simulink model "zaw_int"  (R2013a)
settings: Solver=ode3  StartTime=0.0  StopTime=10.0  FixedStep=0.005  RelTol=1e-3
values from neighbouring files (symbols this model uses):
  c1 = 100    [matlab.mat]    (also in matlab1.mat; matlab3.mat; matlab4.mat)
  c2 = 2000    [matlab.mat]    (also in matlab1.mat; matlab3.mat; matlab4.mat)
  k1 = 370000    [matlab.mat]    (also in matlab1.mat; matlab3.mat; matlab4.mat)
  k2 = 35000    [matlab.mat]    (also in matlab1.mat; matlab3.mat; matlab4.mat = 15000)
  m1 = 90    [matlab.mat]    (also in matlab1.mat; matlab3.mat; matlab4.mat)
  m2 = 600    [matlab.mat]    (also in matlab1.mat; matlab3.mat; matlab4.mat)
  T1 = 0.88    [matlab3.mat]    (also in matlab4.mat)
settings Model: Creator=adasdeb  LastModifiedBy=adasdeb

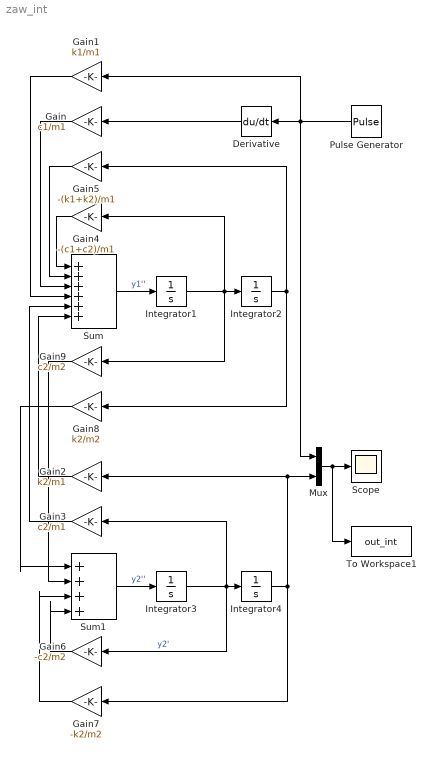
== system zaw_int ==
  Derivative : Derivative
  Gain : Gain  Gain=c1/m1
  Gain1 : Gain  Gain=k1/m1
  Gain2 : Gain  Gain=k2/m1
  Gain3 : Gain  Gain=c2/m1
  Gain4 : Gain  Gain=-(c1+c2)/m1
  Gain5 : Gain  Gain=-(k1+k2)/m1
  Gain6 : Gain  Gain=-c2/m2
  Gain7 : Gain  Gain=-k2/m2
  Gain8 : Gain  Gain=k2/m2
  Gain9 : Gain  Gain=c2/m2
  Integrator{1..4} (4 alike) : Integrator
  Mux : Mux  Inputs=2
  Pulse Generator : DiscretePulseGenerator  PulseType=Time based  Period=T1  PulseWidth=50
  Scope : Scope
      settings: YMin=-2  YMax=2
  Sum : Sum  Inputs=|++++++|
  Sum1 : Sum  Inputs=|++++|
  To Workspace1 : ToWorkspace  VariableName=out_int  SampleTime=-1
  wires:
  Integrator1/1 -> Gain9/1, Integrator2/1, Gain4/1
  Integrator3/1 -> Gain3/1, Gain6/1, Integrator4/1  "y2'"
  Sum/1 -> Integrator1/1  "y1''"
  Sum1/1 -> Integrator3/1  "y2''"
  Gain4/1 -> Sum/1
  Gain5/1 -> Sum/2
  Gain6/1 -> Sum1/4
  Gain7/1 -> Sum1/3
  Gain8/1 -> Sum1/1
  Gain9/1 -> Sum1/2
  Integrator2/1 -> Gain8/1, Gain5/1
  Integrator4/1 -> Gain2/1, Mux/2, Gain7/1
  Mux/1 -> Scope/1, To Workspace1/1
  Gain/1 -> Sum/3
  Gain1/1 -> Sum/4
  Gain2/1 -> Sum/6
  Gain3/1 -> Sum/5
  Derivative/1 -> Gain/1
  Pulse Generator/1 -> Derivative/1, Gain1/1, Mux/1
